simulink model "foc_sim"  (R2024b)
settings: Solver=FixedStepDiscrete  StartTime=0.0  StopTime=10.0  FixedStep=1e-6  RelTol=1e-3
undefined symbols (not defined in the file): B, BW, Flux, J, Ls, Pole_Pairs, Rs, Ts
libraries: slpidlib x3, mcbplantlib x1, autolibpmsmexterior x1
settings Model: Creator=bzwan  LastModifiedBy=bzwan

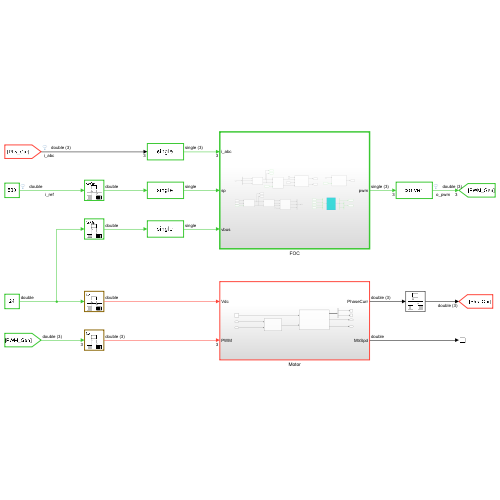
[thumbnail: Simulink's stored preview of the top-level diagram]
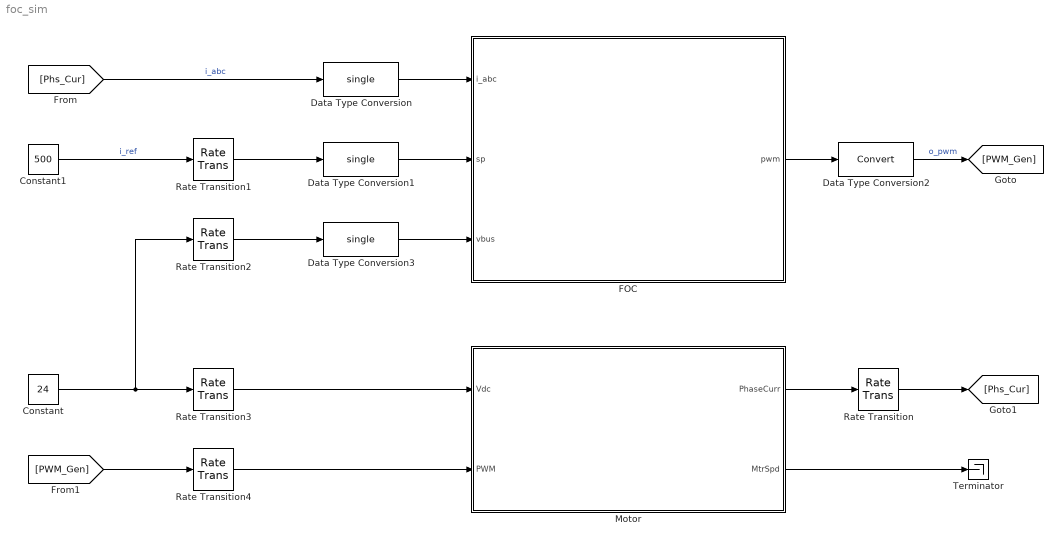
== system foc_sim ==
  Constant : Constant  Value=24  SampleTime=Ts
  Constant1 : Constant  Value=500  SampleTime=Ts
  Data Type Conversion : DataTypeConversion  OutDataTypeStr=single  SaturateOnIntegerOverflow=off  RndMeth=Floor
  Data Type Conversion1 : DataTypeConversion  OutDataTypeStr=single  SaturateOnIntegerOverflow=off  RndMeth=Floor
  Data Type Conversion2 : DataTypeConversion  SaturateOnIntegerOverflow=off  RndMeth=Floor
  Data Type Conversion3 : DataTypeConversion  OutDataTypeStr=single  SaturateOnIntegerOverflow=off  RndMeth=Floor
  FOC : Subsystem  TreatAsAtomicUnit=on  SystemSampleTime=Ts
  Motor : Subsystem
  Rate Transition{,1..4} (5 alike) : RateTransition
  Terminator : Terminator
  wires:
  [Phs_Cur] -> Data Type Conversion/1  "i_abc"
  FOC/1(pwm) -> Data Type Conversion2/1
  Data Type Conversion2/1 -> [PWM_Gen]  "o_pwm"
  Constant1/1 -> Rate Transition1/1  "i_ref"
  [PWM_Gen] -> Rate Transition4/1
  Motor/1(PhaseCurr) -> Rate Transition/1
  Motor/2(MtrSpd) -> Terminator/1
  Data Type Conversion/1 -> FOC/1(i_abc)
  Data Type Conversion1/1 -> FOC/2(sp)
  Data Type Conversion3/1 -> FOC/3(vbus)
  Constant/1 -> Rate Transition2/1, Rate Transition3/1
  Rate Transition1/1 -> Data Type Conversion1/1
  Rate Transition2/1 -> Data Type Conversion3/1
  Rate Transition3/1 -> Motor/1(Vdc)
  Rate Transition4/1 -> Motor/2(PWM)
  Rate Transition/1 -> [Phs_Cur]

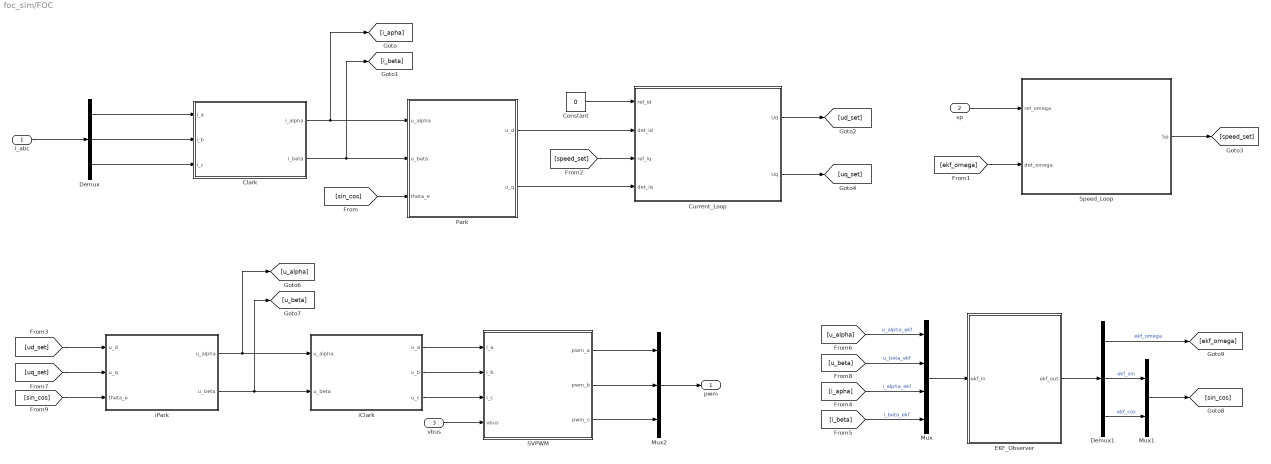
== system foc_sim/FOC ==
  i_abc : Inport
  sp : Inport  Port=2
  vbus : Inport  Port=3
  Clark : MATLAB Function  TreatAsAtomicUnit=on
  Constant : Constant  Value=0  OutDataTypeStr=single  SampleTime=-1
  Current_Loop : Subsystem  TreatAsAtomicUnit=on
  Demux : Demux  Outputs=3
  Demux1 : Demux  Outputs=3
  EKF_Observer : Subsystem
      mask Display:
      | port_label('input',1,'ui_{\alpha\beta}','texmode','on');
      | 
      | port_label('output',1,'\theta_{hat}','texmode','on');
      | 
      | fprintf('EKF_Observer');
  Mux : Mux
  Mux1 : Mux  Inputs=2
  Mux2 : Mux  Inputs=3
  Park : MATLAB Function  TreatAsAtomicUnit=on
  SVPWM : MATLAB Function  TreatAsAtomicUnit=on
  Speed_Loop : Subsystem  TreatAsAtomicUnit=on
  iClark : MATLAB Function  TreatAsAtomicUnit=on
  iPark : MATLAB Function  TreatAsAtomicUnit=on
  pwm : Outport
  wires:
  [i_apha] -> Mux/3  "i_alpha_ekf"
  Demux1/2 -> Mux1/1  "ekf_sin"
  [u_beta] -> Mux/2  "u_beta_ekf"
  EKF_Observer/1(ekf_out) -> Demux1/1
  Mux/1 -> EKF_Observer/1(ekf_in)
  [i_beta] -> Mux/4  "i_beta_ekf"
  [u_alpha] -> Mux/1  "u_alpha_ekf"
  Mux1/1 -> [sin_cos]
  Demux1/1 -> [ekf_omega]  "ekf_omega"
  Demux1/3 -> Mux1/2  "ekf_cos"
  iClark/1(u_a) -> SVPWM/1(i_a)
  iClark/2(u_b) -> SVPWM/2(i_b)
  iClark/3(u_c) -> SVPWM/3(i_c)
  Demux/1 -> Clark/1(i_a)
  Demux/2 -> Clark/2(i_b)
  Demux/3 -> Clark/3(i_c)
  i_abc/1 -> Demux/1
  Clark/1(i_alpha) -> [i_apha], Park/1(u_alpha)
  [sin_cos] -> Park/3(theta_e)
  Clark/2(i_beta) -> Park/2(u_beta), [i_beta]
  Park/1(u_d) -> Current_Loop/2(det_id)
  Park/2(u_q) -> Current_Loop/4(det_iq)
  Constant/1 -> Current_Loop/1(ref_id)
  sp/1 -> Speed_Loop/1(ref_omega)
  [ekf_omega] -> Speed_Loop/2(det_omega)
  Speed_Loop/1(Sp) -> [speed_set]
  [speed_set] -> Current_Loop/3(ref_iq)
  Current_Loop/1(Ud) -> [ud_set]
  Current_Loop/2(Uq) -> [uq_set]
  [ud_set] -> iPark/1(u_d)
  [sin_cos] -> iPark/3(theta_e)
  iPark/1(u_alpha) -> [u_alpha], iClark/1(u_alpha)
  iPark/2(u_beta) -> [u_beta], iClark/2(u_beta)
  SVPWM/1(pwm_a) -> Mux2/1
  SVPWM/2(pwm_b) -> Mux2/2
  SVPWM/3(pwm_c) -> Mux2/3
  [uq_set] -> iPark/2(u_q)
  Mux2/1 -> pwm/1
  vbus/1 -> SVPWM/4(vbus)

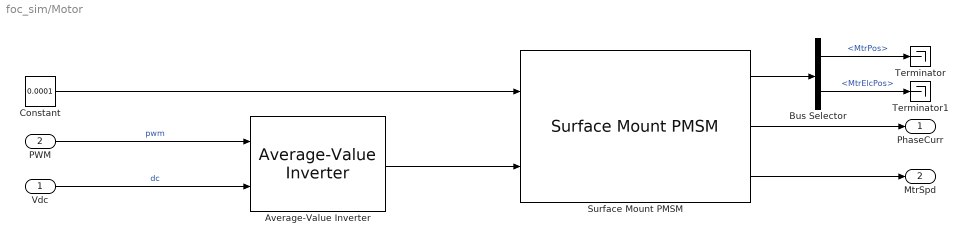
== system foc_sim/Motor ==
  Vdc : Inport
  PWM : Inport  Port=2
  Average-Value Inverter : mcbplantlib/Average-Value Inverter
  Bus Selector : BusSelector  OutputSignals=MtrPos,MtrElcPos
  Constant : Constant  Value=0.0001  SampleTime=-1
  Surface Mount PMSM : autolibpmsmexterior/Surface Mount PMSM  port_config=Torque  sim_type=Discrete  Ts=Ts*0.01  P=Pole_Pairs  Rs=Rs  Ldq_=Ls  KConstText=Permanent flux linkage constant (lambda_pm):  lambda_pm=Flux  Ke=159.9771  Kt=1.323  mechanical=[J, B, 0.01]  idq0=[0 0]  theta_init=0  omega_init=0  KConst=Flux  lambda_pm_calc=Flux  RefBlkName='autolibpmsmexterior/Surface Mount PMSM'  aMode=5  Ldq="[0.0017      0.0017]"
  Terminator : Terminator
  Terminator1 : Terminator
  PhaseCurr : Outport
  MtrSpd : Outport  Port=2
  wires:
  Surface Mount PMSM/1 -> Bus Selector/1
  Vdc/1 -> Average-Value Inverter/2  "dc"
  Constant/1 -> Surface Mount PMSM/1
  Bus Selector/1 -> Terminator/1  "<MtrPos>"
  Bus Selector/2 -> Terminator1/1  "<MtrElcPos>"
  Average-Value Inverter/1 -> Surface Mount PMSM/2
  Surface Mount PMSM/3 -> MtrSpd/1
  PWM/1 -> Average-Value Inverter/1  "pwm"
  Surface Mount PMSM/2 -> PhaseCurr/1

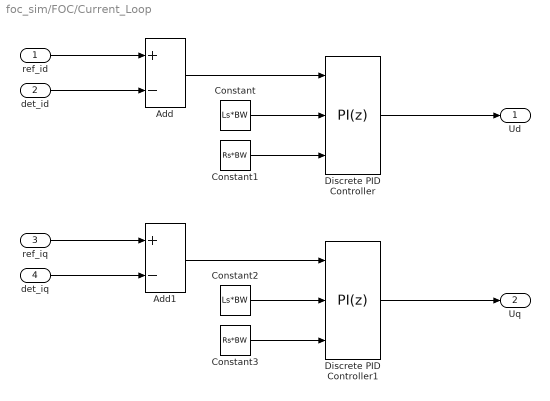
== system foc_sim/FOC/Current_Loop ==
  ref_id : Inport
  det_id : Inport  Port=2
  ref_iq : Inport  Port=3
  det_iq : Inport  Port=4
  Add : Sum  Inputs=+-
  Add1 : Sum  Inputs=+-
  Constant : Constant  Value=Ls*BW  OutDataTypeStr=single  SampleTime=-1
  Constant1 : Constant  Value=Rs*BW  OutDataTypeStr=single  SampleTime=-1
  Constant2 : Constant  Value=Ls*BW  OutDataTypeStr=single  SampleTime=-1
  Constant3 : Constant  Value=Rs*BW  OutDataTypeStr=single  SampleTime=-1
  Discrete PID Controller : slpidlib/PID Controller  Controller=PI  Form=Parallel  TimeDomain=Discrete-time  UseExternalTs=off  SampleTime=-1  IntegratorMethod=Forward Euler  FilterMethod=Forward Euler  ControllerParametersSource=external  P=1  I=1  UseKiTs=off  D=0  UseExternalDerivativeSource=off  N=100  UseFilter=on  TunerSelectOption=Transfer Function Based (PID Tuner App)  InitialConditionSource=internal  InitialConditionForIntegrator=0  InitialConditionForFilter=0  DifferentiatorICPrevScaledInput=0  ExternalReset=none  TrackingMode=off  Kt=1  LimitOutput=off  SatLimitsSource=internal  UpperSaturationLimit=inf  LowerSaturationLimit=-inf  LinearizeAsGain=off  AntiWindupMode=clamping  Kb=1  LimitIntegrator=off  UpperIntegratorSaturationLimit=inf  LowerIntegratorSaturationLimit=-inf  POutMin=[]  POutMax=[]  IOutMin=[]  IOutMax=[]  DOutMin=[]  DOutMax=[]  NOutMin=[]  NOutMax=[]  SumOutMin=[]  SumOutMax=[]  SaturationOutMin=[]  SaturationOutMax=[]  PParamMin=[]  PParamMax=[]  IParamMin=[]  IParamMax=[]  DParamMin=[]  DParamMax=[]  NParamMin=[]  NParamMax=[]  KbParamMin=[]  KbParamMax=[]  KtParamMin=[]  KtParamMax=[]  KbOutMin=[]  KbOutMax=[]  KtOutMin=[]  KtOutMax=[]  IntegratorOutMin=[]  IntegratorOutMax=[]  FilterOutMin=[]  FilterOutMax=[]  SumI1OutMin=[]  SumI1OutMax=[]  SumI2OutMin=[]  SumI2OutMax=[]  SumI3OutMin=[]  SumI3OutMax=[]  SumI4OutMin=[]  SumI4OutMax=[]  SumDOutMin=[]  SumDOutMax=[]  DifferentiatorOutMin=[]  DifferentiatorOutMax=[]  FilterDiffOutCoefMin=[]  FilterDiffOutCoefMax=[]  ReciprocalOutMin=[]  ReciprocalOutMax=[]  SumDenOutMin=[]  SumDenOutMax=[]  SumNumOutMin=[]  SumNumOutMax=[]  DivideOutMin=[]  DivideOutMax=[]  UdiffTsProdOutMin=[]  UdiffTsProdOutMax=[]  NTsProdOutMin=[]  NTsProdOutMax=[]  UintegralTsProdOutMin=[]  UintegralTsProdOutMax=[]  UngainTsProdOutMin=[]  UngainTsProdOutMax=[]  ClampingZeroOutDataTypeStr=Inherit: Inherit via back propagation  ClampingZeroOutMin=[]  ClampingZeroOutMax=[]  FilterDenConstantOutDataTypeStr=Inherit: Inherit via back propagation  FilterDenConstantOutMin=[]  FilterDenConstantOutMax=[]  PCopyOutDataTypeStr=Inherit: Inherit via back propagation  PCopyOutMin=[]  PCopyOutMax=[]  NCopyOutDataTypeStr=Inherit: Inherit via back propagation  NCopyOutMin=[]  NCopyOutMax=[]  IntegratorContinuousStateAttributes=''  IntegratorStateMustResolveToSignalObject=off  IntegratorRTWStateStorageClass=Auto  FilterContinuousStateAttributes=''  FilterStateMustResolveToSignalObject=off  FilterRTWStateStorageClass=Auto  ParallelPVariant=ExternalParameters  IdealPVariant=Disabled  IVariant=ExternalParameters  DVariant=Disabled  IntegratorVariant=Discrete  SatVariant=Disabled  AWVariant=Passthrough  PCopyVariant=Disabled  TRVariant=Disabled  FdbkBlocksVariant=Forward  IdealPFdbkVariant=Disabled  SatFdbkVariant=Disabled  DerivativeFilterVariant=Disabled  NVariant=Disabled  NCopyVariant=Disabled_SignalSpec  FilterICVariant=Disabled  IntegratorICVariant=InternalICs  ExternalResetVariant=Disabled  TRSumVariant=Passthrough  SumFdbkVariant=Disabled  SumVariant=Sum_PI  TsampFilterVariant=InternalTs  TsampNgainVariant=Passthrough  TsampIntegralVariant=Disabled_SignalSpec  ExternalSaturationOutDataTypeStr=Inherit: Same as second input  DerivativeSourceVariant=Disabled  PreIntVariant=InternalPreInt
  Discrete PID Controller1 : slpidlib/PID Controller  Controller=PI  Form=Parallel  TimeDomain=Discrete-time  UseExternalTs=off  SampleTime=-1  IntegratorMethod=Forward Euler  FilterMethod=Forward Euler  ControllerParametersSource=external  P=1  I=1  UseKiTs=off  D=0  UseExternalDerivativeSource=off  N=100  UseFilter=on  TunerSelectOption=Transfer Function Based (PID Tuner App)  InitialConditionSource=internal  InitialConditionForIntegrator=0  InitialConditionForFilter=0  DifferentiatorICPrevScaledInput=0  ExternalReset=none  TrackingMode=off  Kt=1  LimitOutput=off  SatLimitsSource=internal  UpperSaturationLimit=inf  LowerSaturationLimit=-inf  LinearizeAsGain=off  AntiWindupMode=clamping  Kb=1  LimitIntegrator=off  UpperIntegratorSaturationLimit=inf  LowerIntegratorSaturationLimit=-inf  POutMin=[]  POutMax=[]  IOutMin=[]  IOutMax=[]  DOutMin=[]  DOutMax=[]  NOutMin=[]  NOutMax=[]  SumOutMin=[]  SumOutMax=[]  SaturationOutMin=[]  SaturationOutMax=[]  PParamMin=[]  PParamMax=[]  IParamMin=[]  IParamMax=[]  DParamMin=[]  DParamMax=[]  NParamMin=[]  NParamMax=[]  KbParamMin=[]  KbParamMax=[]  KtParamMin=[]  KtParamMax=[]  KbOutMin=[]  KbOutMax=[]  KtOutMin=[]  KtOutMax=[]  IntegratorOutMin=[]  IntegratorOutMax=[]  FilterOutMin=[]  FilterOutMax=[]  SumI1OutMin=[]  SumI1OutMax=[]  SumI2OutMin=[]  SumI2OutMax=[]  SumI3OutMin=[]  SumI3OutMax=[]  SumI4OutMin=[]  SumI4OutMax=[]  SumDOutMin=[]  SumDOutMax=[]  DifferentiatorOutMin=[]  DifferentiatorOutMax=[]  FilterDiffOutCoefMin=[]  FilterDiffOutCoefMax=[]  ReciprocalOutMin=[]  ReciprocalOutMax=[]  SumDenOutMin=[]  SumDenOutMax=[]  SumNumOutMin=[]  SumNumOutMax=[]  DivideOutMin=[]  DivideOutMax=[]  UdiffTsProdOutMin=[]  UdiffTsProdOutMax=[]  NTsProdOutMin=[]  NTsProdOutMax=[]  UintegralTsProdOutMin=[]  UintegralTsProdOutMax=[]  UngainTsProdOutMin=[]  UngainTsProdOutMax=[]  ClampingZeroOutDataTypeStr=Inherit: Inherit via back propagation  ClampingZeroOutMin=[]  ClampingZeroOutMax=[]  FilterDenConstantOutDataTypeStr=Inherit: Inherit via back propagation  FilterDenConstantOutMin=[]  FilterDenConstantOutMax=[]  PCopyOutDataTypeStr=Inherit: Inherit via back propagation  PCopyOutMin=[]  PCopyOutMax=[]  NCopyOutDataTypeStr=Inherit: Inherit via back propagation  NCopyOutMin=[]  NCopyOutMax=[]  IntegratorContinuousStateAttributes=''  IntegratorStateMustResolveToSignalObject=off  IntegratorRTWStateStorageClass=Auto  FilterContinuousStateAttributes=''  FilterStateMustResolveToSignalObject=off  FilterRTWStateStorageClass=Auto  ParallelPVariant=ExternalParameters  IdealPVariant=Disabled  IVariant=ExternalParameters  DVariant=Disabled  IntegratorVariant=Discrete  SatVariant=Disabled  AWVariant=Passthrough  PCopyVariant=Disabled  TRVariant=Disabled  FdbkBlocksVariant=Forward  IdealPFdbkVariant=Disabled  SatFdbkVariant=Disabled  DerivativeFilterVariant=Disabled  NVariant=Disabled  NCopyVariant=Disabled_SignalSpec  FilterICVariant=Disabled  IntegratorICVariant=InternalICs  ExternalResetVariant=Disabled  TRSumVariant=Passthrough  SumFdbkVariant=Disabled  SumVariant=Sum_PI  TsampFilterVariant=InternalTs  TsampNgainVariant=Passthrough  TsampIntegralVariant=Disabled_SignalSpec  ExternalSaturationOutDataTypeStr=Inherit: Same as second input  DerivativeSourceVariant=Disabled  PreIntVariant=InternalPreInt
  Ud : Outport
  Uq : Outport  Port=2
  wires:
  Add/1 -> Discrete PID Controller/1
  Discrete PID Controller1/1 -> Uq/1
  Constant/1 -> Discrete PID Controller/2
  Constant2/1 -> Discrete PID Controller1/2
  det_id/1 -> Add/2
  Constant1/1 -> Discrete PID Controller/3
  Discrete PID Controller/1 -> Ud/1
  Constant3/1 -> Discrete PID Controller1/3
  ref_id/1 -> Add/1
  det_iq/1 -> Add1/2
  Add1/1 -> Discrete PID Controller1/1
  ref_iq/1 -> Add1/1

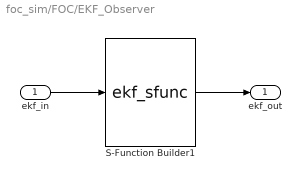
== system foc_sim/FOC/EKF_Observer ==
  ekf_in : Inport
  S-Function Builder1 : S-Function  FunctionName=ekf_sfunc  SFunctionModules=ekf_sfunc_wrapper.c  SFunctionDeploymentMode=off  EnableBusSupport=off  mask(S-Function Builder){}
      mask help: Simulink:masks:SFunctionBuilder_MD
      mask init:
      | val = [[.9  0.75 0.75 1 1 .9 .9 1]',[1 1 0.75 0.75 .9 .9 1 .9]'];try , sys = get_param(gcb,'SfunBuilderFcnName');if isempty(sys), sys = get_param(gcb,'FunctionName'); end,catch, sys = get_param(gcb,'FunctionName'); end
      settings: CopyFcn=set_param(gcbh,'LinkStatus','none')  OpenFcn=sfunctionwizard(gcbh)
      mask Display:
      | plot(val(:,1),val(:,2))
      | disp(sys)
      | port_label('input',1,sprintf('%s', 'u'),'interpreter','tex')
      | port_label('output',1,sprintf('%s', 'y'),'interpreter','tex')
  ekf_out : Outport
  wires:
  S-Function Builder1/1 -> ekf_out/1
  ekf_in/1 -> S-Function Builder1/1

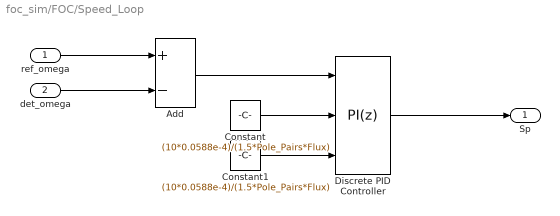
== system foc_sim/FOC/Speed_Loop ==
  ref_omega : Inport
  det_omega : Inport  Port=2
  Add : Sum  Inputs=+-
  Constant : Constant  Value=(10*0.0588e-4)/(1.5*Pole_Pairs*Flux)  OutDataTypeStr=single  SampleTime=-1
  Constant1 : Constant  Value=(10*0.0588e-4)/(1.5*Pole_Pairs*Flux)  OutDataTypeStr=single  SampleTime=-1
  Discrete PID Controller : slpidlib/PID Controller  Controller=PI  Form=Parallel  TimeDomain=Discrete-time  UseExternalTs=off  SampleTime=-1  IntegratorMethod=Forward Euler  FilterMethod=Forward Euler  ControllerParametersSource=external  P=1  I=1  UseKiTs=off  D=0  UseExternalDerivativeSource=off  N=100  UseFilter=on  TunerSelectOption=Transfer Function Based (PID Tuner App)  InitialConditionSource=internal  InitialConditionForIntegrator=0  InitialConditionForFilter=0  DifferentiatorICPrevScaledInput=0  ExternalReset=none  TrackingMode=off  Kt=1  LimitOutput=off  SatLimitsSource=internal  UpperSaturationLimit=inf  LowerSaturationLimit=-inf  LinearizeAsGain=off  AntiWindupMode=clamping  Kb=1  LimitIntegrator=off  UpperIntegratorSaturationLimit=inf  LowerIntegratorSaturationLimit=-inf  POutMin=[]  POutMax=[]  IOutMin=[]  IOutMax=[]  DOutMin=[]  DOutMax=[]  NOutMin=[]  NOutMax=[]  SumOutMin=[]  SumOutMax=[]  SaturationOutMin=[]  SaturationOutMax=[]  PParamMin=[]  PParamMax=[]  IParamMin=[]  IParamMax=[]  DParamMin=[]  DParamMax=[]  NParamMin=[]  NParamMax=[]  KbParamMin=[]  KbParamMax=[]  KtParamMin=[]  KtParamMax=[]  KbOutMin=[]  KbOutMax=[]  KtOutMin=[]  KtOutMax=[]  IntegratorOutMin=[]  IntegratorOutMax=[]  FilterOutMin=[]  FilterOutMax=[]  SumI1OutMin=[]  SumI1OutMax=[]  SumI2OutMin=[]  SumI2OutMax=[]  SumI3OutMin=[]  SumI3OutMax=[]  SumI4OutMin=[]  SumI4OutMax=[]  SumDOutMin=[]  SumDOutMax=[]  DifferentiatorOutMin=[]  DifferentiatorOutMax=[]  FilterDiffOutCoefMin=[]  FilterDiffOutCoefMax=[]  ReciprocalOutMin=[]  ReciprocalOutMax=[]  SumDenOutMin=[]  SumDenOutMax=[]  SumNumOutMin=[]  SumNumOutMax=[]  DivideOutMin=[]  DivideOutMax=[]  UdiffTsProdOutMin=[]  UdiffTsProdOutMax=[]  NTsProdOutMin=[]  NTsProdOutMax=[]  UintegralTsProdOutMin=[]  UintegralTsProdOutMax=[]  UngainTsProdOutMin=[]  UngainTsProdOutMax=[]  ClampingZeroOutDataTypeStr=Inherit: Inherit via back propagation  ClampingZeroOutMin=[]  ClampingZeroOutMax=[]  FilterDenConstantOutDataTypeStr=Inherit: Inherit via back propagation  FilterDenConstantOutMin=[]  FilterDenConstantOutMax=[]  PCopyOutDataTypeStr=Inherit: Inherit via back propagation  PCopyOutMin=[]  PCopyOutMax=[]  NCopyOutDataTypeStr=Inherit: Inherit via back propagation  NCopyOutMin=[]  NCopyOutMax=[]  IntegratorContinuousStateAttributes=''  IntegratorStateMustResolveToSignalObject=off  IntegratorRTWStateStorageClass=Auto  FilterContinuousStateAttributes=''  FilterStateMustResolveToSignalObject=off  FilterRTWStateStorageClass=Auto  ParallelPVariant=ExternalParameters  IdealPVariant=Disabled  IVariant=ExternalParameters  DVariant=Disabled  IntegratorVariant=Discrete  SatVariant=Disabled  AWVariant=Passthrough  PCopyVariant=Disabled  TRVariant=Disabled  FdbkBlocksVariant=Forward  IdealPFdbkVariant=Disabled  SatFdbkVariant=Disabled  DerivativeFilterVariant=Disabled  NVariant=Disabled  NCopyVariant=Disabled_SignalSpec  FilterICVariant=Disabled  IntegratorICVariant=InternalICs  ExternalResetVariant=Disabled  TRSumVariant=Passthrough  SumFdbkVariant=Disabled  SumVariant=Sum_PI  TsampFilterVariant=InternalTs  TsampNgainVariant=Passthrough  TsampIntegralVariant=Disabled_SignalSpec  ExternalSaturationOutDataTypeStr=Inherit: Same as second input  DerivativeSourceVariant=Disabled  PreIntVariant=InternalPreInt
  Sp : Outport
  wires:
  Add/1 -> Discrete PID Controller/1
  Constant/1 -> Discrete PID Controller/2
  det_omega/1 -> Add/2
  Constant1/1 -> Discrete PID Controller/3
  Discrete PID Controller/1 -> Sp/1
  ref_omega/1 -> Add/1

== matlab function foc_sim/FOC/iClark ==
  data: u_alpha input; u_a output; u_beta input; u_b output; u_c output
function [u_a, u_b, u_c] = iclark_fun(u_alpha, u_beta)
%#codegen
    u_a = u_alpha;
    u_b = -1/2*u_alpha + sqrt(3)/2*u_beta;
    u_c = -1/2*u_alpha - sqrt(3)/2*u_beta;
end

== matlab function foc_sim/FOC/Clark ==
  data: i_a input; i_alpha output; i_b input; i_c input; i_beta output
function [i_alpha, i_beta] = clark_fun(i_a, i_b, i_c)
%#codegen
    i_alpha = 2/3*i_a - 1/3*(i_b + i_c);
    i_beta = sqrt(3)/3*(i_b + i_c);
end

== matlab function foc_sim/FOC/Park ==
  data: u_alpha input; u_d output; u_beta input; u_q output; theta_e input
function [u_d, u_q] = park_fun(u_alpha, u_beta, theta_e)
%#codegen
    u_d = u_alpha*theta_e(2) + u_beta*theta_e(1);
    u_q = u_beta*theta_e(2) - u_alpha*theta_e(1);
end

== matlab function foc_sim/FOC/iPark ==
  data: u_d input; u_alpha output; u_q input; theta_e input; u_beta output
function [u_alpha, u_beta] = ipark_fun(u_d, u_q, theta_e)
%#codegen
    u_alpha = u_d*theta_e(2) - u_q*theta_e(1);
    u_beta = u_d*theta_e(1) + u_q*theta_e(2);
end

== matlab function foc_sim/FOC/SVPWM ==
  data: i_a input; pwm_a output; i_b input; pwm_b output; pwm_c output; i_c input; vbus input
function [pwm_a, pwm_b, pwm_c] = svpwm_fun(i_a, i_b, i_c, vbus)
%#codegen
    % mean_zero
    min_val = min([i_a, i_b, i_c]);
    max_val = max([i_a, i_b, i_c]);
    sum_val = min_val + max_val;

    m_zero = -1/2*sum_val;

    % pwm gen
    pwm_a = (i_a + m_zero)/vbus + 0.5;
    pwm_b = (i_b + m_zero)/vbus + 0.5;
    pwm_c = (i_c + m_zero)/vbus + 0.5;
end
